simulink model "P4Simulink"  (R2025b)
settings: Solver=VariableStepAuto  StartTime=0.0  StopTime=10.0  RelTol=1e-3
values from neighbouring files (symbols this model uses):
  k = 100    [P4CodigoSimu.m]
  m = 10    [P4CodigoSimu.m]
  r = 0.05    [P4CodigoSimu.m]
settings Model: Creator=juani  LastModifiedBy=juani

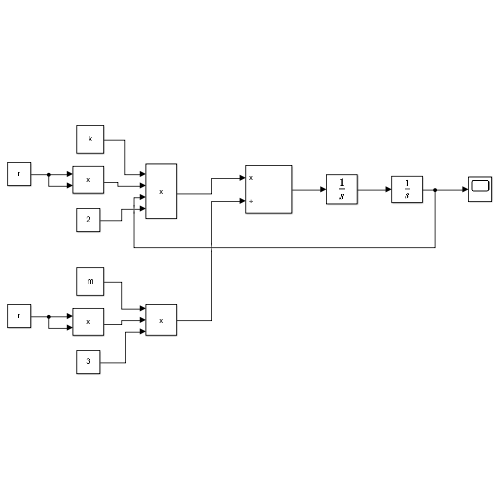
[thumbnail: Simulink's stored preview of the top-level diagram]
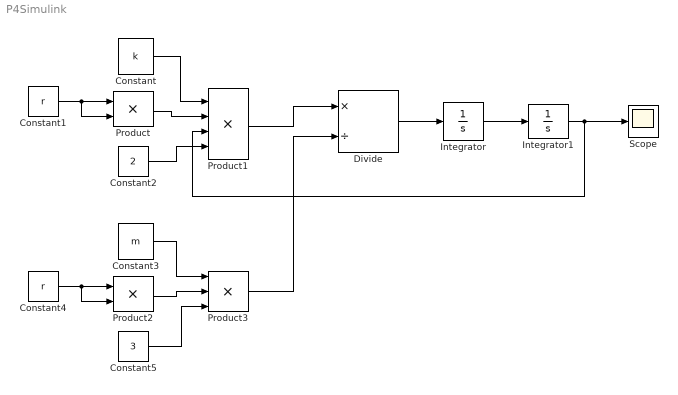
== system P4Simulink ==
  Constant : Constant  Value=k
  Constant1 : Constant  Value=r
  Constant2 : Constant  Value=2
  Constant3 : Constant  Value=m
  Constant4 : Constant  Value=r
  Constant5 : Constant  Value=3
  Divide : Product  Inputs=*/
  Integrator : Integrator  InitialCondition=2
  Integrator1 : Integrator
  Product : Product
  Product1 : Product  Inputs=4
  Product2 : Product
  Product3 : Product  Inputs=3
  Scope : Scope
      settings: ActiveDisplayYMinimum=-1  ActiveDisplayYMaximum=1
  wires:
  Constant1/1 -> Product/2, Product/1
  Constant/1 -> Product1/1
  Product/1 -> Product1/2
  Constant2/1 -> Product1/4
  Constant4/1 -> Product2/2, Product2/1
  Product2/1 -> Product3/2
  Constant5/1 -> Product3/3
  Constant3/1 -> Product3/1
  Product1/1 -> Divide/1
  Product3/1 -> Divide/2
  Divide/1 -> Integrator/1
  Integrator/1 -> Integrator1/1
  Integrator1/1 -> Scope/1, Product1/3
